simulink model "sistema5_4"  (R2025b)
settings: Solver=VariableStepAuto  StartTime=0.0  StopTime=10.0  RelTol=1e-3
libraries: slpidlib x2

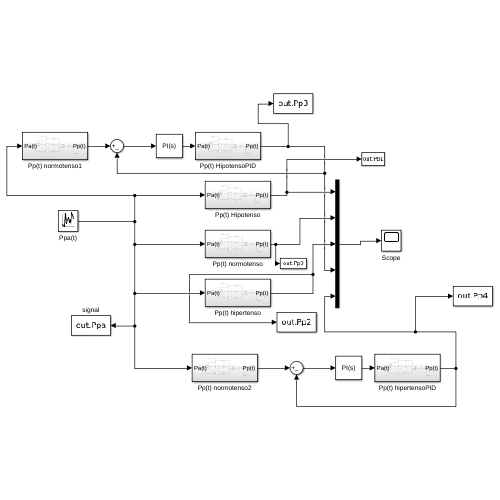
[thumbnail: Simulink's stored preview of the top-level diagram]
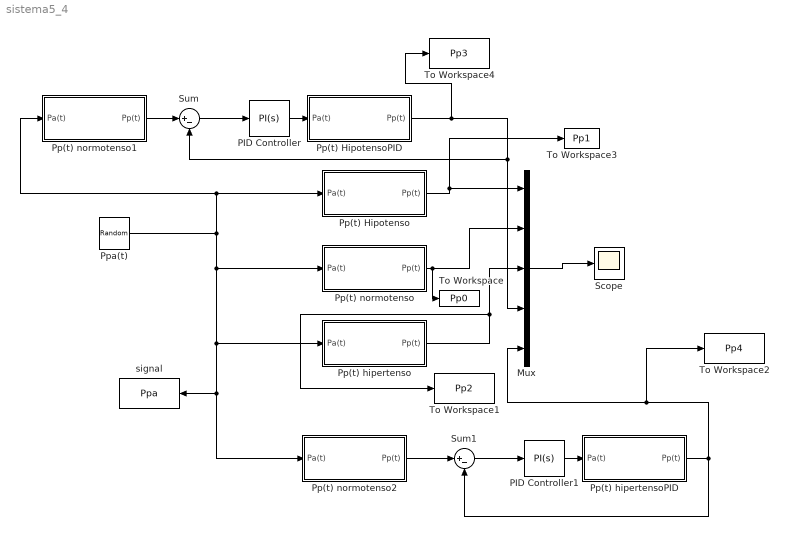
== system sistema5_4 ==
  Mux : Mux  Inputs=5
  PID Controller : slpidlib/PID Controller  Controller=PI  Form=Parallel  TimeDomain=Continuous-time  UseExternalTs=off  SampleTime=-1  IntegratorMethod=Forward Euler  FilterMethod=Forward Euler  ControllerParametersSource=internal  P=4.21636346738391e-05  I=3267.68674685278  UseKiTs=off  D=0  UseExternalDerivativeSource=off  N=100  UseFilter=on  TunerSelectOption=Transfer Function Based (PID Tuner App)  InitialConditionSource=internal  InitialConditionForIntegrator=0  InitialConditionForFilter=0  DifferentiatorICPrevScaledInput=0  ExternalReset=none  TrackingMode=off  Kt=1  LimitOutput=off  SatLimitsSource=internal  UpperSaturationLimit=inf  LowerSaturationLimit=-inf  LinearizeAsGain=on  AntiWindupMode=none  Kb=1  LimitIntegrator=off  UpperIntegratorSaturationLimit=inf  LowerIntegratorSaturationLimit=-inf  POutMin=[]  POutMax=[]  IOutMin=[]  IOutMax=[]  DOutMin=[]  DOutMax=[]  NOutMin=[]  NOutMax=[]  SumOutMin=[]  SumOutMax=[]  SaturationOutMin=[]  SaturationOutMax=[]  PParamMin=[]  PParamMax=[]  IParamMin=[]  IParamMax=[]  DParamMin=[]  DParamMax=[]  NParamMin=[]  NParamMax=[]  KbParamMin=[]  KbParamMax=[]  KtParamMin=[]  KtParamMax=[]  KbOutMin=[]  KbOutMax=[]  KtOutMin=[]  KtOutMax=[]  IntegratorOutMin=[]  IntegratorOutMax=[]  FilterOutMin=[]  FilterOutMax=[]  SumI1OutMin=[]  SumI1OutMax=[]  SumI2OutMin=[]  SumI2OutMax=[]  SumI3OutMin=[]  SumI3OutMax=[]  SumI4OutMin=[]  SumI4OutMax=[]  SumDOutMin=[]  SumDOutMax=[]  DifferentiatorOutMin=[]  DifferentiatorOutMax=[]  FilterDiffOutCoefMin=[]  FilterDiffOutCoefMax=[]  ReciprocalOutMin=[]  ReciprocalOutMax=[]  SumDenOutMin=[]  SumDenOutMax=[]  SumNumOutMin=[]  SumNumOutMax=[]  DivideOutMin=[]  DivideOutMax=[]  UdiffTsProdOutMin=[]  UdiffTsProdOutMax=[]  NTsProdOutMin=[]  NTsProdOutMax=[]  UintegralTsProdOutMin=[]  UintegralTsProdOutMax=[]  UngainTsProdOutMin=[]  UngainTsProdOutMax=[]  ClampingZeroOutDataTypeStr=Inherit: Inherit via back propagation  ClampingZeroOutMin=[]  ClampingZeroOutMax=[]  FilterDenConstantOutDataTypeStr=Inherit: Inherit via back propagation  FilterDenConstantOutMin=[]  FilterDenConstantOutMax=[]  PCopyOutDataTypeStr=Inherit: Inherit via back propagation  PCopyOutMin=[]  PCopyOutMax=[]  NCopyOutDataTypeStr=Inherit: Inherit via back propagation  NCopyOutMin=[]  NCopyOutMax=[]  IntegratorContinuousStateAttributes=''  IntegratorStateMustResolveToSignalObject=off  IntegratorRTWStateStorageClass=Auto  FilterContinuousStateAttributes=''  FilterStateMustResolveToSignalObject=off  FilterRTWStateStorageClass=Auto  ParallelPVariant=InternalParameters  IdealPVariant=Disabled  IVariant=InternalParameters  DVariant=Disabled  IntegratorVariant=Continuous  SatVariant=Disabled  AWVariant=Passthrough  PCopyVariant=Disabled  TRVariant=Disabled  FdbkBlocksVariant=Forward  IdealPFdbkVariant=Disabled  SatFdbkVariant=Disabled  DerivativeFilterVariant=Disabled  NVariant=Disabled  NCopyVariant=Disabled_SignalSpec  FilterICVariant=Disabled  IntegratorICVariant=InternalICs  ExternalResetVariant=Disabled  TRSumVariant=Passthrough  SumFdbkVariant=Disabled  SumVariant=Sum_PI  TsampFilterVariant=InternalTs  TsampNgainVariant=Passthrough  TsampIntegralVariant=Disabled_SignalSpec  ExternalSaturationOutDataTypeStr=Inherit: Same as second input  DerivativeSourceVariant=Disabled  PreIntVariant=InternalPreInt
  PID Controller1 : slpidlib/PID Controller  Controller=PI  Form=Parallel  TimeDomain=Continuous-time  UseExternalTs=off  SampleTime=-1  IntegratorMethod=Forward Euler  FilterMethod=Forward Euler  ControllerParametersSource=internal  P=10  I=31622776.4963  UseKiTs=off  D=0  UseExternalDerivativeSource=off  N=100  UseFilter=on  TunerSelectOption=Transfer Function Based (PID Tuner App)  InitialConditionSource=internal  InitialConditionForIntegrator=0  InitialConditionForFilter=0  DifferentiatorICPrevScaledInput=0  ExternalReset=none  TrackingMode=off  Kt=1  LimitOutput=off  SatLimitsSource=internal  UpperSaturationLimit=inf  LowerSaturationLimit=-inf  LinearizeAsGain=on  AntiWindupMode=none  Kb=1  LimitIntegrator=off  UpperIntegratorSaturationLimit=inf  LowerIntegratorSaturationLimit=-inf  POutMin=[]  POutMax=[]  IOutMin=[]  IOutMax=[]  DOutMin=[]  DOutMax=[]  NOutMin=[]  NOutMax=[]  SumOutMin=[]  SumOutMax=[]  SaturationOutMin=[]  SaturationOutMax=[]  PParamMin=[]  PParamMax=[]  IParamMin=[]  IParamMax=[]  DParamMin=[]  DParamMax=[]  NParamMin=[]  NParamMax=[]  KbParamMin=[]  KbParamMax=[]  KtParamMin=[]  KtParamMax=[]  KbOutMin=[]  KbOutMax=[]  KtOutMin=[]  KtOutMax=[]  IntegratorOutMin=[]  IntegratorOutMax=[]  FilterOutMin=[]  FilterOutMax=[]  SumI1OutMin=[]  SumI1OutMax=[]  SumI2OutMin=[]  SumI2OutMax=[]  SumI3OutMin=[]  SumI3OutMax=[]  SumI4OutMin=[]  SumI4OutMax=[]  SumDOutMin=[]  SumDOutMax=[]  DifferentiatorOutMin=[]  DifferentiatorOutMax=[]  FilterDiffOutCoefMin=[]  FilterDiffOutCoefMax=[]  ReciprocalOutMin=[]  ReciprocalOutMax=[]  SumDenOutMin=[]  SumDenOutMax=[]  SumNumOutMin=[]  SumNumOutMax=[]  DivideOutMin=[]  DivideOutMax=[]  UdiffTsProdOutMin=[]  UdiffTsProdOutMax=[]  NTsProdOutMin=[]  NTsProdOutMax=[]  UintegralTsProdOutMin=[]  UintegralTsProdOutMax=[]  UngainTsProdOutMin=[]  UngainTsProdOutMax=[]  ClampingZeroOutDataTypeStr=Inherit: Inherit via back propagation  ClampingZeroOutMin=[]  ClampingZeroOutMax=[]  FilterDenConstantOutDataTypeStr=Inherit: Inherit via back propagation  FilterDenConstantOutMin=[]  FilterDenConstantOutMax=[]  PCopyOutDataTypeStr=Inherit: Inherit via back propagation  PCopyOutMin=[]  PCopyOutMax=[]  NCopyOutDataTypeStr=Inherit: Inherit via back propagation  NCopyOutMin=[]  NCopyOutMax=[]  IntegratorContinuousStateAttributes=''  IntegratorStateMustResolveToSignalObject=off  IntegratorRTWStateStorageClass=Auto  FilterContinuousStateAttributes=''  FilterStateMustResolveToSignalObject=off  FilterRTWStateStorageClass=Auto  ParallelPVariant=InternalParameters  IdealPVariant=Disabled  IVariant=InternalParameters  DVariant=Disabled  IntegratorVariant=Continuous  SatVariant=Disabled  AWVariant=Passthrough  PCopyVariant=Disabled  TRVariant=Disabled  FdbkBlocksVariant=Forward  IdealPFdbkVariant=Disabled  SatFdbkVariant=Disabled  DerivativeFilterVariant=Disabled  NVariant=Disabled  NCopyVariant=Disabled_SignalSpec  FilterICVariant=Disabled  IntegratorICVariant=InternalICs  ExternalResetVariant=Disabled  TRSumVariant=Passthrough  SumFdbkVariant=Disabled  SumVariant=Sum_PI  TsampFilterVariant=InternalTs  TsampNgainVariant=Passthrough  TsampIntegralVariant=Disabled_SignalSpec  ExternalSaturationOutDataTypeStr=Inherit: Same as second input  DerivativeSourceVariant=Disabled  PreIntVariant=InternalPreInt
  Pp(t) Hipotenso : Subsystem
  Pp(t) HipotensoPID : Subsystem
  Pp(t) hipertenso : Subsystem
  Pp(t) hipertensoPID : Subsystem
  Pp(t) normotenso : Subsystem
  Pp(t) normotenso1 : Subsystem
  Pp(t) normotenso2 : Subsystem
  Ppa(t) : UniformRandomNumber  Minimum=-0.2  Seed=106  SampleTime=0.5
  Scope : Scope
      settings: ActiveDisplayYMinimum=-0.31887216328582157  ActiveDisplayYMaximum=1.1949397115901816
  Sum : Sum  Inputs=|+-
  Sum1 : Sum  Inputs=|+-
  To Workspace : ToWorkspace  VariableName=Pp0  SampleTime=-1
      settings: Save2DSignal=2-D array (concatenate along first dimension)
  To Workspace1 : ToWorkspace  VariableName=Pp2  SampleTime=-1
      settings: Save2DSignal=2-D array (concatenate along first dimension)
  To Workspace2 : ToWorkspace  VariableName=Pp4  SampleTime=-1
      settings: Save2DSignal=2-D array (concatenate along first dimension)
  To Workspace3 : ToWorkspace  VariableName=Pp1  SampleTime=-1
      settings: Save2DSignal=2-D array (concatenate along first dimension)
  To Workspace4 : ToWorkspace  VariableName=Pp3  SampleTime=-1
      settings: Save2DSignal=2-D array (concatenate along first dimension)
  signal : ToWorkspace  VariableName=Ppa  SampleTime=-1
      settings: Save2DSignal=2-D array (concatenate along first dimension)
  wires:
  Pp(t) hipertenso/1(Pp(t)) -> To Workspace1/1, Mux/3
  Pp(t) normotenso/1(Pp(t)) -> Mux/2, To Workspace/1
  Mux/1 -> Scope/1
  Pp(t) Hipotenso/1(Pp(t)) -> To Workspace3/1, Mux/1
  Ppa(t)/1 -> Pp(t) Hipotenso/1(Pa(t)), Pp(t) normotenso1/1(Pa(t)), signal/1, Pp(t) normotenso2/1(Pa(t)), Pp(t) hipertenso/1(Pa(t)), Pp(t) normotenso/1(Pa(t))
  Pp(t) normotenso1/1(Pp(t)) -> Sum/1
  Sum/1 -> PID Controller/1
  PID Controller/1 -> Pp(t) HipotensoPID/1(Pa(t))
  Pp(t) HipotensoPID/1(Pp(t)) -> To Workspace4/1, Sum/2, Mux/4
  Sum1/1 -> PID Controller1/1
  PID Controller1/1 -> Pp(t) hipertensoPID/1(Pa(t))
  Pp(t) normotenso2/1(Pp(t)) -> Sum1/1
  Pp(t) hipertensoPID/1(Pp(t)) -> To Workspace2/1, Mux/5, Sum1/2

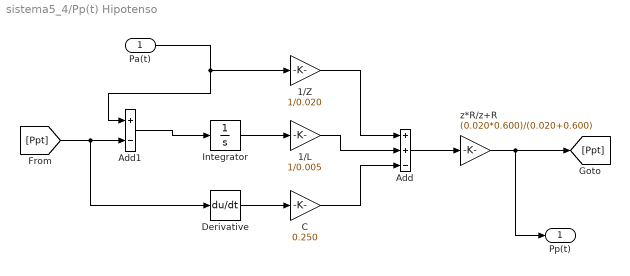
== system sistema5_4/Pp(t) Hipotenso ==
  Pa(t) : Inport
  1/L : Gain  Gain=1/0.005
  1/Z : Gain  Gain=1/0.020
  Add : Sum  Inputs=++-
  Add1 : Sum  Inputs=+-
  C : Gain  Gain=0.250
  Derivative : Derivative
  Integrator : Integrator
  z*R/z+R : Gain  Gain=(0.020*0.600)/(0.020+0.600)
  Pp(t) : Outport
  wires:
  1/Z/1 -> Add/1
  1/L/1 -> Add/2
  C/1 -> Add/3
  Add/1 -> z*R/z+R/1
  Pa(t)/1 -> Add1/1, 1/Z/1
  Derivative/1 -> C/1
  Integrator/1 -> 1/L/1
  z*R/z+R/1 -> [Ppt], Pp(t)/1
  Add1/1 -> Integrator/1
  [Ppt] -> Derivative/1, Add1/2

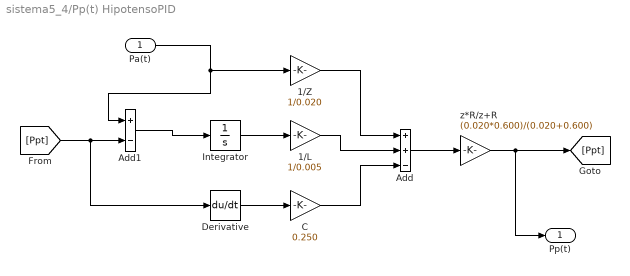
== system sistema5_4/Pp(t) HipotensoPID ==
  Pa(t) : Inport
  1/L : Gain  Gain=1/0.005
  1/Z : Gain  Gain=1/0.020
  Add : Sum  Inputs=++-
  Add1 : Sum  Inputs=+-
  C : Gain  Gain=0.250
  Derivative : Derivative
  Integrator : Integrator
  z*R/z+R : Gain  Gain=(0.020*0.600)/(0.020+0.600)
  Pp(t) : Outport
  wires:
  1/Z/1 -> Add/1
  1/L/1 -> Add/2
  C/1 -> Add/3
  Add/1 -> z*R/z+R/1
  Pa(t)/1 -> Add1/1, 1/Z/1
  Derivative/1 -> C/1
  Integrator/1 -> 1/L/1
  z*R/z+R/1 -> [Ppt], Pp(t)/1
  Add1/1 -> Integrator/1
  [Ppt] -> Derivative/1, Add1/2

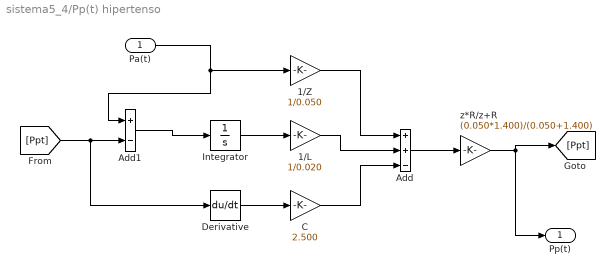
== system sistema5_4/Pp(t) hipertenso ==
  Pa(t) : Inport
  1/L : Gain  Gain=1/0.020
  1/Z : Gain  Gain=1/0.050
  Add : Sum  Inputs=++-
  Add1 : Sum  Inputs=+-
  C : Gain  Gain=2.500
  Derivative : Derivative
  Integrator : Integrator
  z*R/z+R : Gain  Gain=(0.050*1.400)/(0.050+1.400)
  Pp(t) : Outport
  wires:
  1/Z/1 -> Add/1
  1/L/1 -> Add/2
  C/1 -> Add/3
  Add/1 -> z*R/z+R/1
  Pa(t)/1 -> Add1/1, 1/Z/1
  Derivative/1 -> C/1
  Integrator/1 -> 1/L/1
  z*R/z+R/1 -> [Ppt], Pp(t)/1
  Add1/1 -> Integrator/1
  [Ppt] -> Derivative/1, Add1/2

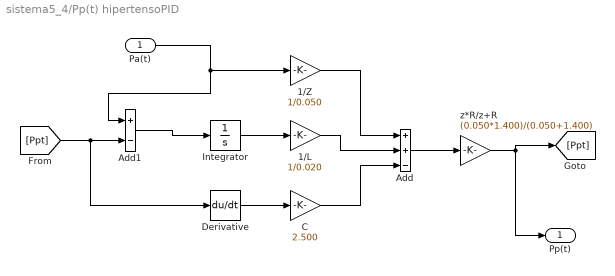
== system sistema5_4/Pp(t) hipertensoPID ==
  Pa(t) : Inport
  1/L : Gain  Gain=1/0.020
  1/Z : Gain  Gain=1/0.050
  Add : Sum  Inputs=++-
  Add1 : Sum  Inputs=+-
  C : Gain  Gain=2.500
  Derivative : Derivative
  Integrator : Integrator
  z*R/z+R : Gain  Gain=(0.050*1.400)/(0.050+1.400)
  Pp(t) : Outport
  wires:
  1/Z/1 -> Add/1
  1/L/1 -> Add/2
  C/1 -> Add/3
  Add/1 -> z*R/z+R/1
  Pa(t)/1 -> Add1/1, 1/Z/1
  Derivative/1 -> C/1
  Integrator/1 -> 1/L/1
  z*R/z+R/1 -> [Ppt], Pp(t)/1
  Add1/1 -> Integrator/1
  [Ppt] -> Derivative/1, Add1/2

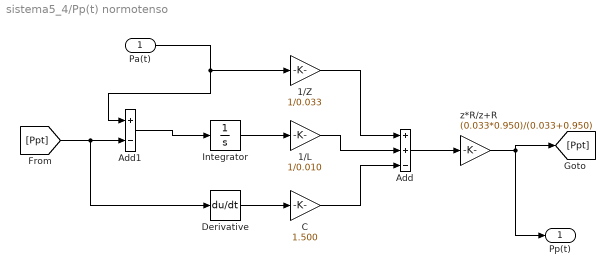
== system sistema5_4/Pp(t) normotenso ==
  Pa(t) : Inport
  1/L : Gain  Gain=1/0.010
  1/Z : Gain  Gain=1/0.033
  Add : Sum  Inputs=++-
  Add1 : Sum  Inputs=+-
  C : Gain  Gain=1.500
  Derivative : Derivative
  Integrator : Integrator
  z*R/z+R : Gain  Gain=(0.033*0.950)/(0.033+0.950)
  Pp(t) : Outport
  wires:
  1/Z/1 -> Add/1
  1/L/1 -> Add/2
  C/1 -> Add/3
  Add/1 -> z*R/z+R/1
  Pa(t)/1 -> Add1/1, 1/Z/1
  Derivative/1 -> C/1
  Integrator/1 -> 1/L/1
  z*R/z+R/1 -> [Ppt], Pp(t)/1
  Add1/1 -> Integrator/1
  [Ppt] -> Derivative/1, Add1/2

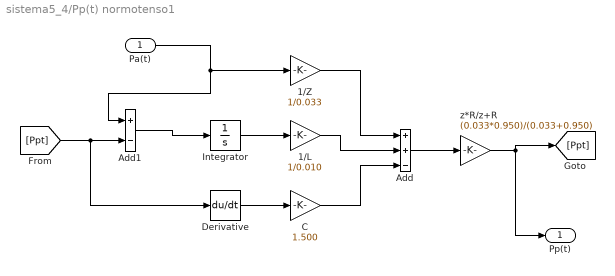
== system sistema5_4/Pp(t) normotenso1 ==
  Pa(t) : Inport
  1/L : Gain  Gain=1/0.010
  1/Z : Gain  Gain=1/0.033
  Add : Sum  Inputs=++-
  Add1 : Sum  Inputs=+-
  C : Gain  Gain=1.500
  Derivative : Derivative
  Integrator : Integrator
  z*R/z+R : Gain  Gain=(0.033*0.950)/(0.033+0.950)
  Pp(t) : Outport
  wires:
  1/Z/1 -> Add/1
  1/L/1 -> Add/2
  C/1 -> Add/3
  Add/1 -> z*R/z+R/1
  Pa(t)/1 -> Add1/1, 1/Z/1
  Derivative/1 -> C/1
  Integrator/1 -> 1/L/1
  z*R/z+R/1 -> [Ppt], Pp(t)/1
  Add1/1 -> Integrator/1
  [Ppt] -> Derivative/1, Add1/2

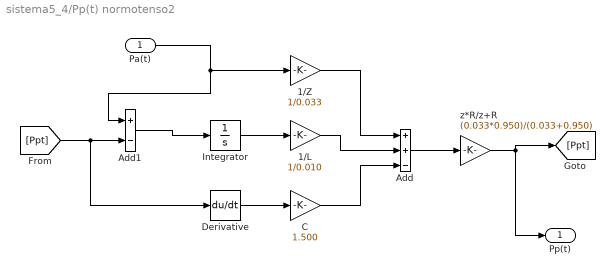
== system sistema5_4/Pp(t) normotenso2 ==
  Pa(t) : Inport
  1/L : Gain  Gain=1/0.010
  1/Z : Gain  Gain=1/0.033
  Add : Sum  Inputs=++-
  Add1 : Sum  Inputs=+-
  C : Gain  Gain=1.500
  Derivative : Derivative
  Integrator : Integrator
  z*R/z+R : Gain  Gain=(0.033*0.950)/(0.033+0.950)
  Pp(t) : Outport
  wires:
  1/Z/1 -> Add/1
  1/L/1 -> Add/2
  C/1 -> Add/3
  Add/1 -> z*R/z+R/1
  Pa(t)/1 -> Add1/1, 1/Z/1
  Derivative/1 -> C/1
  Integrator/1 -> 1/L/1
  z*R/z+R/1 -> [Ppt], Pp(t)/1
  Add1/1 -> Integrator/1
  [Ppt] -> Derivative/1, Add1/2
